simulink model "soru1"  (R2025b)
settings: Solver=VariableStepAuto  StartTime=0.0  StopTime=30  RelTol=1e-3
settings Model: Creator=Seyma  LastModifiedBy=Seyma

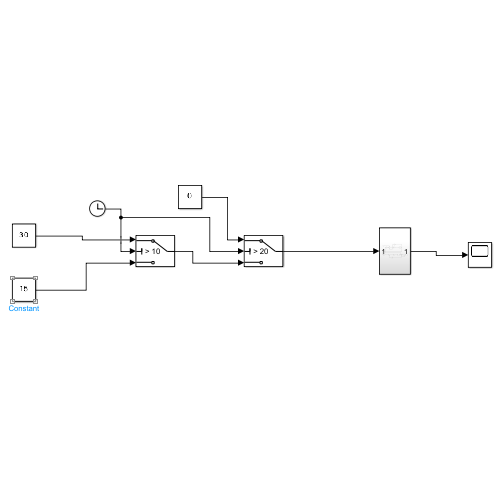
[thumbnail: Simulink's stored preview of the top-level diagram]
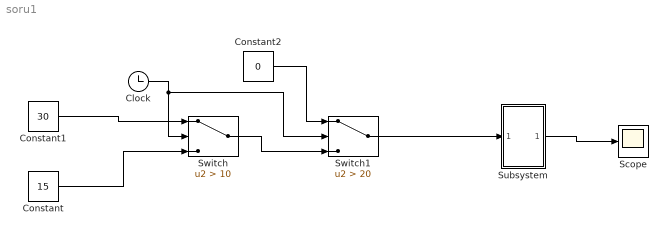
== system soru1 ==
  Clock : Clock
  Constant : Constant  Value=15
  Constant1 : Constant  Value=30
  Constant2 : Constant  Value=0
  Scope : Scope
      settings: ActiveDisplayYMinimum=-3.0737704870609157  ActiveDisplayYMaximum=27.663934383548249
  Subsystem : Subsystem
  Switch : Switch  Criteria=u2 > Threshold  Threshold=10  SaturateOnIntegerOverflow=off  InputSameDT=off
  Switch1 : Switch  Criteria=u2 > Threshold  Threshold=20  SaturateOnIntegerOverflow=off  InputSameDT=off
  wires:
  Clock/1 -> Switch1/2, Switch/2
  Constant1/1 -> Switch/1
  Constant/1 -> Switch/3
  Switch/1 -> Switch1/3
  Constant2/1 -> Switch1/1
  Switch1/1 -> Subsystem/1(In1)
  Subsystem/1(Out1) -> Scope/1

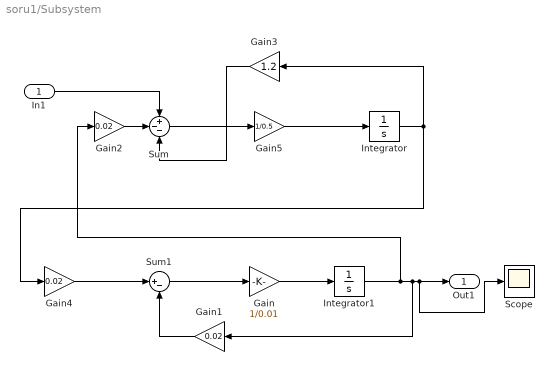
== system soru1/Subsystem ==
  In1 : Inport
  Gain : Gain  Gain=1/0.01
  Gain1 : Gain  Gain=0.02
  Gain2 : Gain  Gain=0.02
  Gain3 : Gain  Gain=1.2
  Gain4 : Gain  Gain=0.02
  Gain5 : Gain  Gain=1/0.5
  Integrator : Integrator
  Integrator1 : Integrator
  Scope : Scope
      settings: ActiveDisplayYMinimum=-1  ActiveDisplayYMaximum=1
  Sum : Sum  Inputs=+--
  Sum1 : Sum  Inputs=|+-
  Out1 : Outport
  wires:
  Gain2/1 -> Sum/2
  Sum1/1 -> Gain/1
  Gain5/1 -> Integrator/1
  Integrator/1 -> Gain3/1, Gain4/1
  Gain3/1 -> Sum/3
  Gain1/1 -> Sum1/2
  Sum/1 -> Gain5/1
  Integrator1/1 -> Gain2/1, Gain1/1, Out1/1, Scope/1
  Gain/1 -> Integrator1/1
  Gain4/1 -> Sum1/1
  In1/1 -> Sum/1
